simulink library "mfeval_LIB"  (R2017b)
settings: Solver=ode45  StartTime=0.0  StopTime=10.0  RelTol=1e-3
undefined symbols (not defined in the file): dynamics, flipSide, parameterStruct, useMode, userDynamics, userUseMode
libraries: mfeval_CPI_LIB x2, mfeval_STI_LIB x2
settings Model: Creator=MFURLANT  LastModifiedBy=MFURLANT
settings DataIOCC: SaveFormat=StructureWithTime
settings OptimizationCC: LifeSpan=inf
settings DebuggingCC: SFExecutionAtInitializationDiag=none
settings HardwareCC: ProdBitPerSizeT=32  ProdBitPerPtrDiffT=32  ProdWordSize=32  ProdHWDeviceType=Specified
settings CodeAppCC: StateflowObjectComments=on
settings GRTTargetCC: TargetLangStandard=C89/C90 (ANSI)

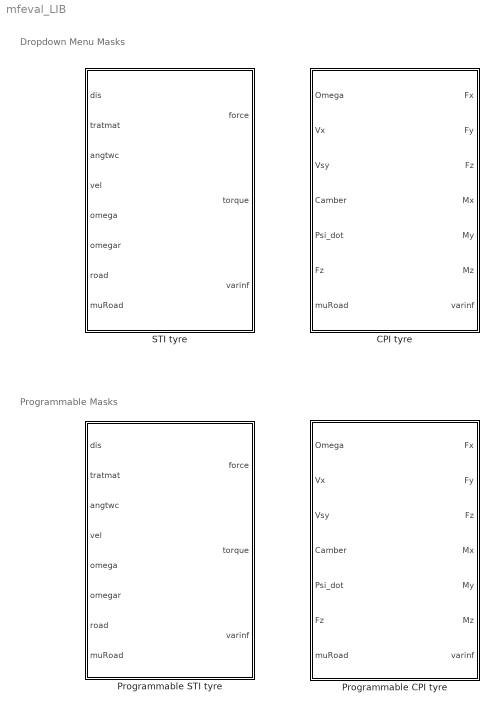
== system mfeval_LIB ==
  note: Dropdown Menu Masks
  note: Programmable Masks
  CPI tyre : Subsystem  Description=Magic Formula 6.1.2 tyre model including relaxation length and transient calculations  TreatAsAtomicUnit=on  mask(mfeval_CPI_tyre){userParameterSource='MagicFormula61_Paramerters.tir', userSide=1 left, userDynamics=3 non-linear transients, userUseMode=1 combined, enablePressure=off, userPressure=2.3}
      mask prompts: userParameterSource "TIR File (String or Structure)"; userSide "Tyre side     :"; userDynamics "Dynamics     :"; userUseMode "Use mode    :"; enablePressure "Set custom Inflation Pressure (bar)"
      mask help:
      | MFeval model using the contact point interface (CPI).
      | Inputs to the model are the sliding velocities at the tyre-road contact point.
      | Forces and Moments are calculated at the tyre-road contact point using a W-axis system.
      mask init:
      | % Check if userParameterSource is a string
      | if(ischar(userParameterSource))
      |     tempParamStruct = mfeval.readTIR(userParameterSource); % Call readTIR function to read the TIR file and obtain a structure of parameters
      | elseif(isstruct(userParameterSource))
      |     tempParamStruct = userParameterSource; % The user has already passed a structure of parameters
      | end
      | 
      | % Check tir file side if field exists
      | if isfield(tempParamStruct, 'TYRESIDE')
      |     if strfind(upper(tempParamStruct.TYRESIDE),'LEFT')
      |         tirFileSide = 1; % 1 is equal to left
      |     else
      |         tirFileSide = 2; % 2 is equal to right
      |     end
      | else
      |     % Default value
      |     tirFileSide = 2; % 2 is equal to right
      | end
      | 
      | % Create a variable to fip the forces depending on the tire side
      | if isequal(tirFileSide, userSide)
      |     flipSide = 0; % No need to flip the tire, user has specified the same side as in the TIR file
      | else
      |     flipSide = 1; % The user has specified a different tire side from the TIR file
      | end
      | 
      | % Keep only the numetic fields (avoir Simulink errors) nd save it into parameterStruct
      | fn = fieldnames(tempParamStruct);
      | for k = 1:numel(fn)
      |     v = tempParamStruct.(fn{k});
      |     if(isnumeric(v))
      |         parameterStruct.(fn{k}) = v;
      |     end
      | end
      mask Help: web( [fullfile(mfevalroot, '..', 'doc','simulinkCPI.html')])
      mask TypeOptions userSide: 1 left | 2 right
      mask TypeOptions userDynamics: 1 steady state | 2 linear transients | 3 non-linear transients
      mask TypeOptions userUseMode: 1 combined | 2 combined+turnslip
      mask Callback enablePressure:
      | % Use the dialog callback to set the
      | % enabling and visibility of parameters
      | 
      | % Get the value of the Enable Pressure checkbox
      | % unchecked = 'off'
      | % checked = 'on'
      | enab = get_param(gcb,'enablePressure');
      | 
      | % Set the 'MaskVisililities' property for each parameters
      | if strcmp(enab,'on')
      |     set_param(gcb,'MaskEnables',{'on','on','on','on','on','on'});
      | else
      |     set_param(gcb,'MaskEnables',{'on','on','on','on','on','off'});
      | end
      | 
      | % Note that the value of the bias is not handled here.
      | % See the Initialization tab
      mask Display: image('TyreLogo.png')
  Programmable CPI tyre : Subsystem  Description=Magic Formula 6.1.2 tyre model including relaxation length and transient calculations  TreatAsAtomicUnit=on  mask(mfeval_CPI_tyre){parameterStruct=parameterStruct, flipSide=flipSide, userDynamics=dynamics, userUseMode=useMode, enablePressure=off, userPressure=2.3}
      mask prompts: parameterStruct "TIR Structure (numeric only)"; flipSide "FlipSide (0=No or  1=Yes)"; userDynamics "Dynamics (1=steady state, 2=linear trans or 3=non-linear trans)"; userUseMode "Use mode (1=combined or 2=comb+turnslip)"; enablePressure "Set custom Inflation Pressure (bar)"
      mask help:
      | MFeval model using the contact point interface (CPI).
      | Inputs to the model are the sliding velocities at the tyre-road contact point.
      | Forces and Moments are calculated at the tyre-road contact point using a W-axis system.
      mask Help: web( [fullfile(mfevalroot, '..', 'doc','simulinkCPI.html')])
      mask Callback enablePressure:
      | % Use the dialog callback to set the
      | % enabling and visibility of parameters
      | 
      | % Get the value of the Enable Pressure checkbox
      | % unchecked = 'off'
      | % checked = 'on'
      | enab = get_param(gcb,'enablePressure');
      | 
      | % Set the 'MaskVisililities' property for each parameters
      | if strcmp(enab,'on')
      |     set_param(gcb,'MaskEnables',{'on','on','on','on','on','on'});
      | else
      |     set_param(gcb,'MaskEnables',{'on','on','on','on','on','off'});
      | end
      | 
      | % Note that the value of the bias is not handled here.
      | % See the Initialization tab
      mask Display: image('TyreLogo.png')
  "Programmable STI tyre " : Subsystem  mask(mfeval_STI_tyre){parameterStruct=parameterStruct, flipSide=flipSide, userDynamics=userDynamics, userUseMode=userUseMode, enablePressure=off, userPressure=2.3}
      mask prompts: parameterStruct "TIR Structure (numeric only)"; flipSide "FlipSide (0=No or  1=Yes)"; userDynamics "Dynamics (1=steady state, 2=linear trans or 3=non-linear trans)"; userUseMode "Use mode (1=combined or 2=comb+turnslip)"; enablePressure "Set custom Inflation Pressure (bar)"
      mask help:
      | MFeval model using the standard tire interface (STI) defined by the TYDEX group.
      | The inputs to the model are the motions at the wheel centre using a C-axis system
      | The model calculates forces and moments at the wheel centre.
      mask Help: web( [fullfile(mfevalroot, '..', 'doc','simulinkSTI.html')])
      mask Callback enablePressure:
      | % Use the dialog callback to set the
      | % enabling and visibility of parameters
      | 
      | % Get the value of the Enable Pressure checkbox
      | % unchecked = 'off'
      | % checked = 'on'
      | enab = get_param(gcb,'enablePressure');
      | 
      | % Set the 'MaskVisililities' property for each parameters
      | if strcmp(enab,'on')
      |     set_param(gcb,'MaskEnables',{'on','on','on','on','on','on'});
      | else
      |     set_param(gcb,'MaskEnables',{'on','on','on','on','on','off'});
      | end
      | 
      | % Note that the value of the bias is not handled here.
      | % See the Initialization tab
      mask Display: image('TyreLogo.png')
  STI tyre : Subsystem  Description=Magic Formula 6.1.2 tyre model including relaxation length and transient calculations  TreatAsAtomicUnit=on  mask(mfeval_STI_tyre){userParameterSource='MagicFormula61_Paramerters.tir', userSide=1 left, userDynamics=2 linear transients, userUseMode=1 combined, enablePressure=off, userPressure=2.3}
      mask prompts: userParameterSource "TIR File (String or Structure)"; userSide "Tyre side      :"; userDynamics "Dynamics     :"; userUseMode "Use mode    :"; enablePressure "Set custom Inflation Pressure (bar)"
      mask help:
      | MFeval model using the standard tire interface (STI) defined by the TYDEX group.
      | The inputs to the model are the motions at the wheel centre using a C-axis system
      | The model calculates forces and moments at the wheel centre.
      mask init: same as mfeval_LIB/CPI tyre
      mask Help: web( [fullfile(mfevalroot, '..', 'doc','simulinkSTI.html')])
      mask TypeOptions userSide: 1 left | 2 right
      mask TypeOptions userDynamics: 1 steady state | 2 linear transients | 3 non-linear transients
      mask TypeOptions userUseMode: 1 combined | 2 combined+turnslip
      mask Callback enablePressure:
      | % Use the dialog callback to set the
      | % enabling and visibility of parameters
      | 
      | % Get the value of the Enable Pressure checkbox
      | % unchecked = 'off'
      | % checked = 'on'
      | enab = get_param(gcb,'enablePressure');
      | 
      | % Set the 'MaskVisililities' property for each parameters
      | if strcmp(enab,'on')
      |     set_param(gcb,'MaskEnables',{'on','on','on','on','on','on'});
      | else
      |     set_param(gcb,'MaskEnables',{'on','on','on','on','on','off'});
      | end
      | 
      | % Note that the value of the bias is not handled here.
      | % See the Initialization tab
      mask Display: image('TyreLogo.png')

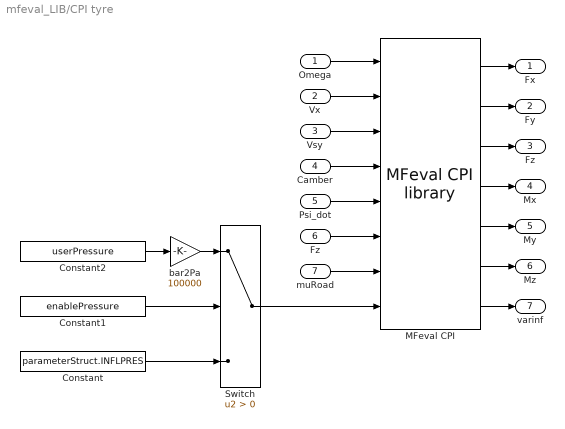
== system mfeval_LIB/CPI tyre ==
  Omega : Inport
  Vx : Inport  Port=2
  Vsy : Inport  Port=3
  Camber : Inport  Port=4
  Psi_dot : Inport  Port=5
  Fz : Inport  Port=6
  muRoad : Inport  Port=7
  Constant : Constant  Value=parameterStruct.INFLPRES
  Constant1 : Constant  Value=enablePressure
  Constant2 : Constant  Value=userPressure
  MFeval CPI : mfeval_CPI_LIB/MFeval CPI library
  Switch : Switch  Criteria=u2 > Threshold
  bar2Pa : Gain  Gain=100000
  Fx : Outport
  Fy : Outport  Port=2
  "Fz " : Outport  Port=3
  Mx : Outport  Port=4
  My : Outport  Port=5
  Mz : Outport  Port=6
  varinf : Outport  Port=7
  wires:
  Vsy/1 -> MFeval CPI/3
  MFeval CPI/5 -> My/1
  Omega/1 -> MFeval CPI/1
  MFeval CPI/1 -> Fx/1
  MFeval CPI/2 -> Fy/1
  Vx/1 -> MFeval CPI/2
  MFeval CPI/3 -> "Fz "/1
  MFeval CPI/4 -> Mx/1
  MFeval CPI/6 -> Mz/1
  MFeval CPI/7 -> varinf/1
  Camber/1 -> MFeval CPI/4
  Psi_dot/1 -> MFeval CPI/5
  Fz/1 -> MFeval CPI/6
  muRoad/1 -> MFeval CPI/7
  Switch/1 -> MFeval CPI/8
  Constant/1 -> Switch/3
  Constant1/1 -> Switch/2
  Constant2/1 -> bar2Pa/1
  bar2Pa/1 -> Switch/1

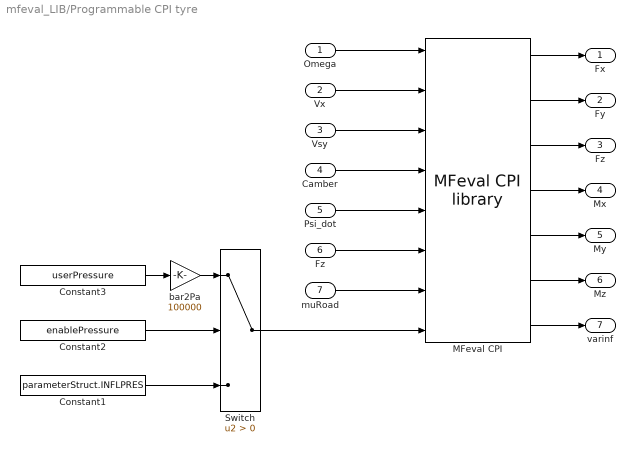
== system mfeval_LIB/Programmable CPI tyre ==
  Omega : Inport
  Vx : Inport  Port=2
  Vsy : Inport  Port=3
  Camber : Inport  Port=4
  Psi_dot : Inport  Port=5
  Fz : Inport  Port=6
  muRoad : Inport  Port=7
  Constant1 : Constant  Value=parameterStruct.INFLPRES
  Constant2 : Constant  Value=enablePressure
  Constant3 : Constant  Value=userPressure
  MFeval CPI : mfeval_CPI_LIB/MFeval CPI library
  Switch : Switch  Criteria=u2 > Threshold
  bar2Pa : Gain  Gain=100000
  Fx : Outport
  Fy : Outport  Port=2
  "Fz " : Outport  Port=3
  Mx : Outport  Port=4
  My : Outport  Port=5
  Mz : Outport  Port=6
  varinf : Outport  Port=7
  wires:
  Camber/1 -> MFeval CPI/4
  Omega/1 -> MFeval CPI/1
  Vsy/1 -> MFeval CPI/3
  Vx/1 -> MFeval CPI/2
  Psi_dot/1 -> MFeval CPI/5
  Fz/1 -> MFeval CPI/6
  MFeval CPI/7 -> varinf/1
  MFeval CPI/6 -> Mz/1
  MFeval CPI/5 -> My/1
  MFeval CPI/4 -> Mx/1
  MFeval CPI/3 -> "Fz "/1
  MFeval CPI/2 -> Fy/1
  MFeval CPI/1 -> Fx/1
  muRoad/1 -> MFeval CPI/7
  Switch/1 -> MFeval CPI/8
  Constant3/1 -> bar2Pa/1
  bar2Pa/1 -> Switch/1
  Constant2/1 -> Switch/2
  Constant1/1 -> Switch/3

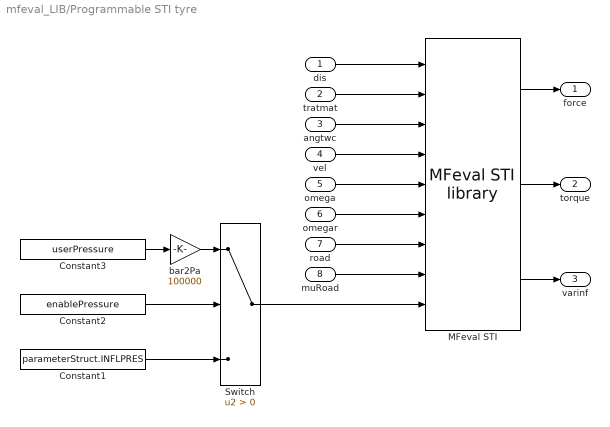
== system mfeval_LIB/Programmable STI tyre  ==
  dis : Inport
  tratmat : Inport  Port=2
  angtwc : Inport  Port=3
  vel : Inport  Port=4
  omega : Inport  Port=5
  omegar : Inport  Port=6
  road : Inport  Port=7
  muRoad : Inport  Port=8
  Constant1 : Constant  Value=parameterStruct.INFLPRES
  Constant2 : Constant  Value=enablePressure
  Constant3 : Constant  Value=userPressure
  MFeval STI : mfeval_STI_LIB/MFeval STI library
  Switch : Switch  Criteria=u2 > Threshold
  bar2Pa : Gain  Gain=100000
  force : Outport
  torque : Outport  Port=2
  varinf : Outport  Port=3
  wires:
  vel/1 -> MFeval STI/4
  omega/1 -> MFeval STI/5
  angtwc/1 -> MFeval STI/3
  road/1 -> MFeval STI/7
  tratmat/1 -> MFeval STI/2
  MFeval STI/2 -> torque/1
  omegar/1 -> MFeval STI/6
  MFeval STI/3 -> varinf/1
  dis/1 -> MFeval STI/1
  MFeval STI/1 -> force/1
  muRoad/1 -> MFeval STI/8
  Switch/1 -> MFeval STI/9
  Constant3/1 -> bar2Pa/1
  bar2Pa/1 -> Switch/1
  Constant2/1 -> Switch/2
  Constant1/1 -> Switch/3

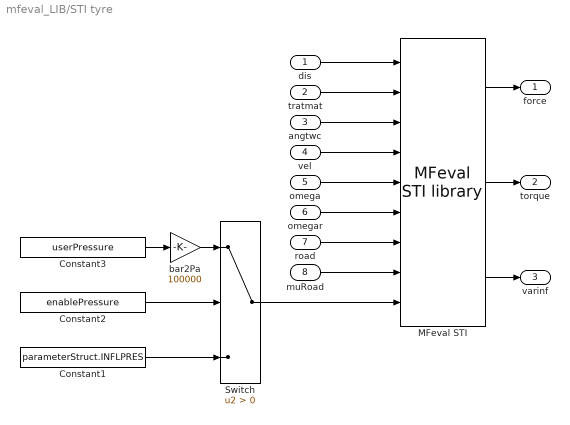
== system mfeval_LIB/STI tyre ==
  dis : Inport
  tratmat : Inport  Port=2
  angtwc : Inport  Port=3
  vel : Inport  Port=4
  omega : Inport  Port=5
  omegar : Inport  Port=6
  road : Inport  Port=7
  muRoad : Inport  Port=8
  Constant1 : Constant  Value=parameterStruct.INFLPRES
  Constant2 : Constant  Value=enablePressure
  Constant3 : Constant  Value=userPressure
  MFeval STI : mfeval_STI_LIB/MFeval STI library
  Switch : Switch  Criteria=u2 > Threshold
  bar2Pa : Gain  Gain=100000
  force : Outport
  torque : Outport  Port=2
  varinf : Outport  Port=3
  wires:
  MFeval STI/2 -> torque/1
  dis/1 -> MFeval STI/1
  tratmat/1 -> MFeval STI/2
  MFeval STI/3 -> varinf/1
  omega/1 -> MFeval STI/5
  angtwc/1 -> MFeval STI/3
  vel/1 -> MFeval STI/4
  MFeval STI/1 -> force/1
  road/1 -> MFeval STI/7
  omegar/1 -> MFeval STI/6
  muRoad/1 -> MFeval STI/8
  Switch/1 -> MFeval STI/9
  Constant3/1 -> bar2Pa/1
  Constant2/1 -> Switch/2
  bar2Pa/1 -> Switch/1
  Constant1/1 -> Switch/3
